simulink model "LgrstCloseLStateCtrl"  (R2018b)
settings: Solver=FixedStepDiscrete  StartTime=0.0  StopTime=10.0  FixedStep=0.01  RelTol=1e-3
libraries: StateCtrlLib x1
settings Model: Creator=sn2xws  LastModifiedBy=sn2xws
settings DataIOCC: SaveFormat=StructureWithTime
settings OptimizationCC: DefaultParameterBehavior=Inlined  EnhancedBackFolding=on  PassReuseOutputArgsAs=Individual arguments  ZeroExternalMemoryAtStartup=off  ZeroInternalMemoryAtStartup=off  OptimizeBlockOrder=speed  DifferentSizesBufferReuse=on  OptimizationCustomize=off
settings DebuggingCC: ParameterTunabilityLossMsg=error
settings ModelReferenceCC: ModelReferenceNumInstancesAllowed=Single
settings SFSimCC: MATLABDynamicMemAlloc=off
settings RTWCC: SystemTargetFile=autosar.tlc  GenCodeOnly=on  TemplateMakefile=ert_default_tmf  Description=AUTOSAR  GenerateReport=on  IncludeHyperlinkInReport=on  LaunchReport=on  GenerateTraceInfo=on  GenerateTraceReport=on  GenerateTraceReportSl=on  GenerateTraceReportSf=on  GenerateTraceReportEml=on
settings CodeAppCC: ForceParamTrailComments=on  IgnoreCustomStorageClasses=off  OperatorAnnotations=on  SimulinkDataObjDesc=on  SFDataObjDesc=on  InsertBlockDesc=on
settings STFCustomTargetCC: TargetLangStandard=C99 (ISO)  MultiwordLength=256  ParMdlRefBuildCompliant=on  CompOptLevelCompliant=on  IncludeMdlTerminateFcn=off  CombineOutputUpdateFcns=on  SuppressErrorStatus=on  ERTCustomFileBanners=on  SupportNonFinite=off  SupportComplex=off  SupportContinuousTime=off  SupportNonInlinedSFcns=off  RemoveResetFunc=on  MATLABClassNameForMDSCustomization=Simulink.SoftwareTarget.ERTCustomization  AutosarCompliant=on  UseToolchainInfoCompliant=on  LookupTableObjectStructAxisOrder=2,1,3,4,...  LUTObjectStructOrderEvenSpacing=Size,Table,Breakpoints  SystemTargetFile=autosar.tlc
settings ERTTargetCC: TargetLangStandard=C99 (ISO)  ConcurrentExecutionCompliant=off  IncludeMdlTerminateFcn=off  SuppressErrorStatus=on  SupportNonFinite=off  SupportComplex=off  ModelStepFunctionPrototypeControlCompliant=off  CPPClassGenCompliant=off  AutosarCompliant=on  LookupTableObjectStructAxisOrder=2,1,3,4,...  LUTObjectStructOrderEvenSpacing=Size,Table,Breakpoints  InlinedParameterPlacement=NonHierarchical  ERTCustomFileTemplate=example_file_process.tlc

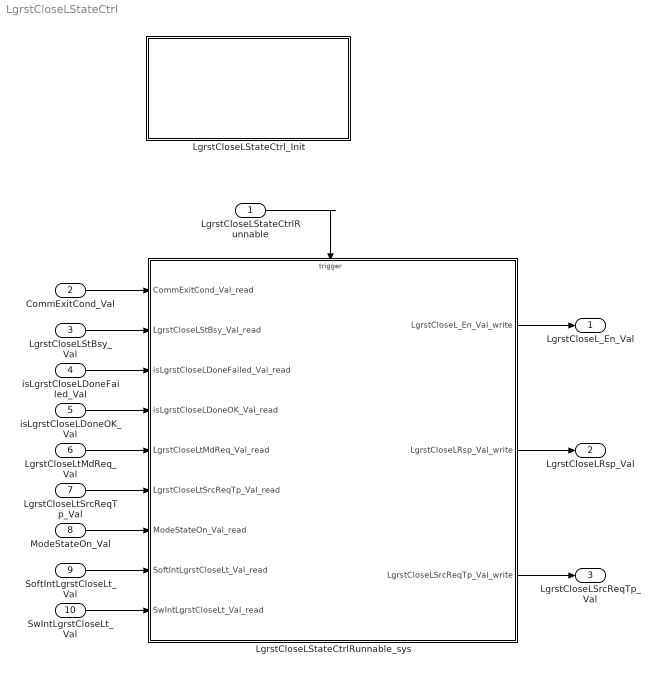
== system LgrstCloseLStateCtrl ==
  LgrstCloseLStateCtrlRunnable : Inport  SampleTime=0.01  OutputFunctionCall=on
  CommExitCond_Val : Inport  Port=2  OutDataTypeStr=boolean  PortDimensions=1
  LgrstCloseLStBsy_Val : Inport  Port=3  OutDataTypeStr=boolean  PortDimensions=1
  isLgrstCloseLDoneFailed_Val : Inport  Port=4  OutDataTypeStr=boolean  PortDimensions=1
  isLgrstCloseLDoneOK_Val : Inport  Port=5  OutDataTypeStr=boolean  PortDimensions=1
  LgrstCloseLtMdReq_Val : Inport  Port=6  OutDataTypeStr=boolean  PortDimensions=1
  LgrstCloseLtSrcReqTp_Val : Inport  Port=7  OutDataTypeStr=Enum: SrcReqTp1  PortDimensions=1
  ModeStateOn_Val : Inport  Port=8  OutDataTypeStr=boolean  PortDimensions=1
  SoftIntLgrstCloseLt_Val : Inport  Port=9  OutDataTypeStr=IntEnable  PortDimensions=1
  SwIntLgrstCloseLt_Val : Inport  Port=10  OutDataTypeStr=IntEnable  PortDimensions=1
  LgrstCloseLStateCtrlRunnable_sys : Subsystem
  LgrstCloseLStateCtrl_Init : Subsystem
  LgrstCloseL_En_Val : Outport  OutDataTypeStr=boolean  PortDimensions=1
  LgrstCloseLRsp_Val : Outport  Port=2  OutDataTypeStr=Enum: MdRspLocal1  PortDimensions=1
  LgrstCloseLSrcReqTp_Val : Outport  Port=3  OutDataTypeStr=Enum: SrcReqTp1  PortDimensions=1
  wires:
  CommExitCond_Val/1 -> LgrstCloseLStateCtrlRunnable_sys/1(CommExitCond_Val_read)
  LgrstCloseLStBsy_Val/1 -> LgrstCloseLStateCtrlRunnable_sys/2(LgrstCloseLStBsy_Val_read)
  isLgrstCloseLDoneFailed_Val/1 -> LgrstCloseLStateCtrlRunnable_sys/3(isLgrstCloseLDoneFailed_Val_read)
  isLgrstCloseLDoneOK_Val/1 -> LgrstCloseLStateCtrlRunnable_sys/4(isLgrstCloseLDoneOK_Val_read)
  LgrstCloseLtMdReq_Val/1 -> LgrstCloseLStateCtrlRunnable_sys/5(LgrstCloseLtMdReq_Val_read)
  LgrstCloseLtSrcReqTp_Val/1 -> LgrstCloseLStateCtrlRunnable_sys/6(LgrstCloseLtSrcReqTp_Val_read)
  ModeStateOn_Val/1 -> LgrstCloseLStateCtrlRunnable_sys/7(ModeStateOn_Val_read)
  SoftIntLgrstCloseLt_Val/1 -> LgrstCloseLStateCtrlRunnable_sys/8(SoftIntLgrstCloseLt_Val_read)
  SwIntLgrstCloseLt_Val/1 -> LgrstCloseLStateCtrlRunnable_sys/9(SwIntLgrstCloseLt_Val_read)
  LgrstCloseLStateCtrlRunnable_sys/1(LgrstCloseL_En_Val_write) -> LgrstCloseL_En_Val/1
  LgrstCloseLStateCtrlRunnable_sys/2(LgrstCloseLRsp_Val_write) -> LgrstCloseLRsp_Val/1
  LgrstCloseLStateCtrlRunnable_sys/3(LgrstCloseLSrcReqTp_Val_write) -> LgrstCloseLSrcReqTp_Val/1
  LgrstCloseLStateCtrlRunnable/1 -> LgrstCloseLStateCtrlRunnable_sys/Trigger

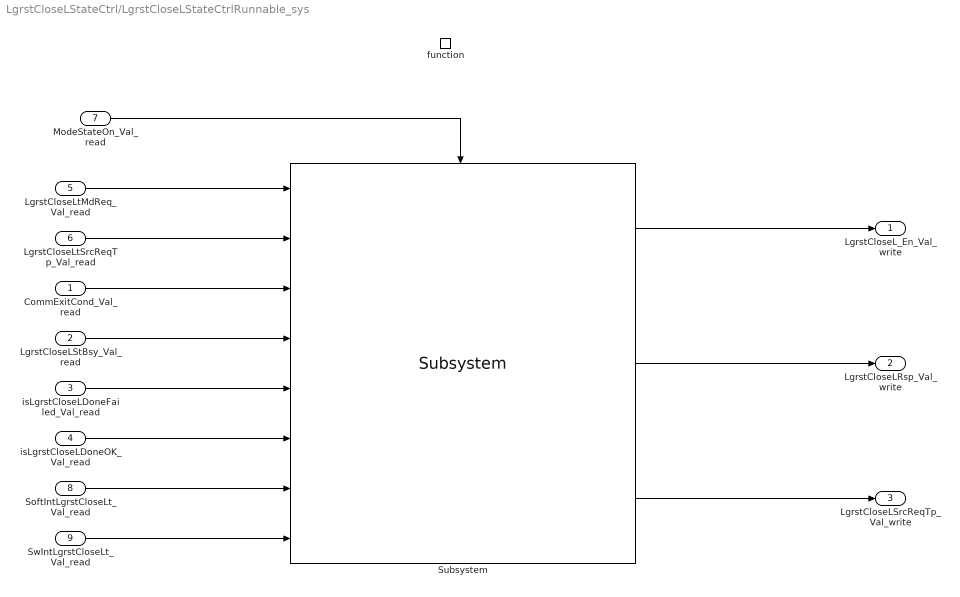
== system LgrstCloseLStateCtrl/LgrstCloseLStateCtrlRunnable_sys ==
  CommExitCond_Val_read : Inport
  LgrstCloseLStBsy_Val_read : Inport  Port=2
  isLgrstCloseLDoneFailed_Val_read : Inport  Port=3
  isLgrstCloseLDoneOK_Val_read : Inport  Port=4
  LgrstCloseLtMdReq_Val_read : Inport  Port=5
  LgrstCloseLtSrcReqTp_Val_read : Inport  Port=6
  ModeStateOn_Val_read : Inport  Port=7
  SoftIntLgrstCloseLt_Val_read : Inport  Port=8
  SwIntLgrstCloseLt_Val_read : Inport  Port=9
  function : TriggerPort  TriggerType=function-call  VariantControl=(inherit)  SampleTimeType=periodic  SampleTime=-1
  Subsystem : StateCtrlLib/Subsystem  SystemSampleTime=-1
  LgrstCloseL_En_Val_write : Outport
      settings: EnsureOutportIsVirtual=on
  LgrstCloseLRsp_Val_write : Outport  Port=2
      settings: EnsureOutportIsVirtual=on
  LgrstCloseLSrcReqTp_Val_write : Outport  Port=3
      settings: EnsureOutportIsVirtual=on
  wires:
  Subsystem/1 -> LgrstCloseL_En_Val_write/1
  Subsystem/2 -> LgrstCloseLRsp_Val_write/1
  Subsystem/3 -> LgrstCloseLSrcReqTp_Val_write/1
  ModeStateOn_Val_read/1 -> Subsystem/Enable
  LgrstCloseLtMdReq_Val_read/1 -> Subsystem/1
  SoftIntLgrstCloseLt_Val_read/1 -> Subsystem/7
  LgrstCloseLtSrcReqTp_Val_read/1 -> Subsystem/2
  CommExitCond_Val_read/1 -> Subsystem/3
  SwIntLgrstCloseLt_Val_read/1 -> Subsystem/8
  LgrstCloseLStBsy_Val_read/1 -> Subsystem/4
  isLgrstCloseLDoneFailed_Val_read/1 -> Subsystem/5
  isLgrstCloseLDoneOK_Val_read/1 -> Subsystem/6

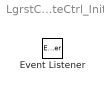
== system LgrstCloseLStateCtrl/LgrstCloseLStateCtrl_Init ==
  Event Listener : EventListener  EventName=reset
